simulink model "feedback_control"  (R2020b)
settings: Solver=FixedStepDiscrete  StartTime=0.0  StopTime=10.0  FixedStep=T_sample_control  RelTol=1e-3  EnableMultiTasking=on
undefined symbols (not defined in the file): T_sample_control
settings Model: DataDictionary=pid.sldd  EnableAccessToBaseWorkspace=off  ModifiedByFormat=The MathWorks Inc.  Creator=The MathWorks, Inc.  LastModifiedBy=The MathWorks Inc.
settings DataIOCC: SaveFormat=Array  ReturnWorkspaceOutputs=off
settings OptimizationCC: DefaultParameterBehavior=Inlined  InlineInvariantSignals=on  PassReuseOutputArgsAs=Individual arguments  ExpressionDepthLimit=2147483647  EfficientFloat2IntCast=on  LifeSpan=1  EfficientTunableParamExpr=on
settings DebuggingCC: SolverPrmCheckMsg=warning  FcnCallInpInsideContextMsg=warning  UniqueDataStoreMsg=error  AssertControl=DisableAll  AllowSymbolicDim=off  StateNameClashWarn=warning  StrictBusMsg=ErrorOnBusTreatedAsVector  SFUnexpectedBacktrackingDiag=warning  SFNoUnconditionalDefaultTransitionDiag=warning  SFExecutionAtInitializationDiag=none  ArithmeticOperatorsInVariantConditions=warning
settings HardwareCC: ProdBitPerPointer=32  ProdBitPerSizeT=32  ProdBitPerPtrDiffT=32  ProdLargestAtomicInteger=Long  ProdLargestAtomicFloat=Double  ProdWordSize=32  ProdHWDeviceType=ARM Compatible->ARM Cortex-M
settings ModelReferenceCC: PropagateSignalLabelsOutOfModel=off
settings SFSimCC: SimUseLocalCustomCode=off  CustomCodeUndefinedFunction=UseInterfaceOnly
settings RTWCC: Description=Embedded Coder  SystemTargetFile=ert.tlc  GenCodeOnly=on  TemplateMakefile=ert_default_tmf  GenerateReport=on  RTWUseLocalCustomCode=off  IncludeHyperlinkInReport=on  GenerateTraceInfo=on  GenerateTraceReport=on  GenerateTraceReportSl=on  GenerateTraceReportSf=on  GenerateTraceReportEml=on  GenerateCodeMetricsReport=on
settings CodeAppCC: IgnoreCustomStorageClasses=off  IgnoreTestpoints=on  CustomSymbolStrType=$N$R$M  StateflowObjectComments=on  InternalIdentifier=Classic
settings ERTTargetCC: MultiwordLength=2048  GenerateSampleERTMain=on  CodeInterfacePackaging=Reusable function  SupportNonFinite=off  ParenthesesLevel=Maximum  InlinedParameterPlacement=NonHierarchical  ERTCustomFileTemplate=example_file_process.tlc  ERTFilePackagingFormat=Compact  ConvertIfToSwitch=off  SuppressUnreachableDefaultCases=off
settings ConfigComp: CovMetricSettings=dw  CovSaveCumulativeToWorkspaceVar=on  CovSaveSingleToWorkspaceVar=on  CovExternalEMLEnable=off  CovSFcnEnable=off

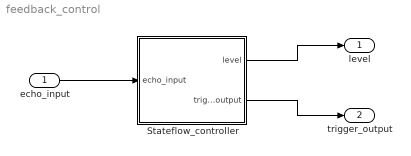
== system feedback_control ==
  echo_input : Inport  OutDataTypeStr=uint8  PortDimensions=1  SampleTime=T_sample_control
  Stateflow_controller : Stateflow chart  TreatAsAtomicUnit=on
  level : Outport  OutDataTypeStr=uint8  PortDimensions=1  SampleTime=T_sample_control
  trigger_output : Outport  Port=2  OutDataTypeStr=uint8
  wires:
  echo_input/1 -> Stateflow_controller/1(echo_input)
  Stateflow_controller/1(level) -> level/1
  Stateflow_controller/2(trigger_output) -> trigger_output/1

== stateflow chart feedback_control/Stateflow_controller ==
  state TRIGGER [parallel]
    settings: executionOrder=1
    state TRIGGER_ON
      en:
      trigger_output=1;
    state TRIGGER_OFF
      en:
      trigger_output=0;
    (default) -> TRIGGER_ON
    TRIGGER_OFF -> TRIGGER_ON : after(60, msec)
    TRIGGER_ON -> TRIGGER_OFF : after(10, usec)
  state LOGIC_OPERATOR [parallel]
    settings: executionOrder=2
    state INITIAL_STATE
      en:
      dist_v=[0 0 0 0]';
      i=1;
      counter=0;
      mean=0;
    state COUNTER
      en,du:
      counter= counter + 1;
    state ERROR
      en:
      up=0.5;
      down=0.5;
    state SAVE_MEASURE
      en:
      dist_v(i)=counter;
    state MEAN
      en:
      mean=(dist_v(1)+dist_v(2)+dist_v(3)+dist_v(4))/232;
      dist_v(1)=dist_v(2);
      dist_v(2)=dist_v(3);
      dist_v(3)=dist_v(4);
      i=4;
    state OUT_RANGE
      en:
      up=0.25;
      down=0.25;
    state IN_RANGE
      en:
      up=(mean*0.001);
      down=(0.1-up);
    (default) -> INITIAL_STATE
    (junction 45) -> INITIAL_STATE
    ERROR -> (junction 45)
    INITIAL_STATE -> (junction 48) [order 2] : after(0.06001, sec)
    (junction 48) -> ERROR
    INITIAL_STATE -> COUNTER [order 1] : [echo_input==1]
    (junction 32) -> COUNTER
    (junction 31) -> (junction 32)
    SAVE_MEASURE -> COUNTER [order 2] : [echo_input==1]{counter=0, i=i+1}
    COUNTER -> SAVE_MEASURE : [echo_input == 0]
    SAVE_MEASURE -> ERROR [order 3] : after(0.06001, sec)
    SAVE_MEASURE -> MEAN [order 1] : [i==4]
    (junction 41) -> ERROR
    MEAN -> IN_RANGE [order 1] : [mean>=10 && mean<=100]
    MEAN -> OUT_RANGE [order 2]
    OUT_RANGE -> (junction 31) [order 1] : [echo_input==1]{counter=0}
    OUT_RANGE -> (junction 36) [order 2] : after(0.06001, sec)
    IN_RANGE -> (junction 31) [order 1] : [echo_input==1]{counter=0}
    IN_RANGE -> (junction 38) [order 2] : after(0.06001, sec)
    (junction 38) -> (junction 41)
    (junction 36) -> (junction 38)
  state LED [parallel]
    settings: executionOrder=3
    state OFF
      en:
      level=0;
    state ON
      en:
      level=1;
    (default) -> OFF
    ON -> OFF : after(up, sec)[down]
    OFF -> ON : after(down, sec)
  data: echo_input input uint8; level output uint8; trigger_output output uint8; counter local uint16; mean local double; i local uint8; dist_v local double; up local double =2; down local double =2
